simulink library "Radiator_basic"  (R2016b)
settings: Solver=ode45  StartTime=0.0  StopTime=10.0  RelTol=1e-3  EnableMultiTasking=on
libraries: carnot x2, simulink_extras x1
settings Model: Creator=drhf  LastModifiedBy=drhf
settings DataIOCC: LimitDataPoints=on  SaveFormat=Array  SignalLoggingSaveFormat=ModelDataLogs
settings OptimizationCC: ExpressionDepthLimit=2147483647  LifeSpan=inf
settings DebuggingCC: UnderspecifiedInitializationDetection=Classic  MergeDetectMultiDrivingBlocksExec=none  SolverPrmCheckMsg=warning  FcnCallInpInsideContextMsg=warning  StateNameClashWarn=warning  SFUnexpectedBacktrackingDiag=warning  SFNoUnconditionalDefaultTransitionDiag=warning  SFExecutionAtInitializationDiag=none
settings HardwareCC: ProdBitPerPointer=32  ProdBitPerSizeT=32  ProdBitPerPtrDiffT=32  ProdLargestAtomicFloat=None  ProdIntDivRoundTo=Undefined  ProdEndianess=Unspecified  ProdWordSize=32  ProdHWDeviceType=32-bit Generic
settings ModelReferenceCC: PropagateSignalLabelsOutOfModel=off
settings GRTTargetCC: TargetLangStandard=C89/C90 (ANSI)  GeneratePreprocessorConditionals=Disable all  CombineOutputUpdateFcns=off  GRTInterface=on
settings ConfigComp: CovMetricSettings=dw  CovHtmlReporting=on  CovSaveCumulativeToWorkspaceVar=on  CovSaveSingleToWorkspaceVar=on  CovExternalEMLEnable=off

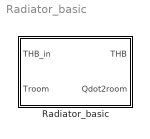
== system Radiator_basic ==
  Radiator_basic : Subsystem  mask(basic Radiator){pnomEN=1000, dtnomEN=50, expo=1.3, mcp=4182*1, tini=20}
      mask prompts: pnomEN "Qdot_nom: nominal power in W"; dtnomEN "Tdiff_nom: nominal temperature difference in K"; expo "radiator exponent (> 0)"; mcp "mass * capacity per unit in J/K"; tini "Initial temperature in °C"
      mask help:
      | The block calculates the heat transfer of a radiator to a room according to the EN 442 equation.
      | Qdot = Qdot_nom * (Tdiff/Tdiff_nom)^n
      mask init:
      | mcap = max(1,mcp); % lower limit for capacity is 1 J/K
      | 
      | % correct values because current model 
      | % uses outlet temperature as mean temperature
      | pnom = pnomEN;
      | dtnom = dtnomEN-5;
      mask Help: web(['file:///' fullfile(path_carnot('help'),'Radiator.html')],'-helpbrowser')

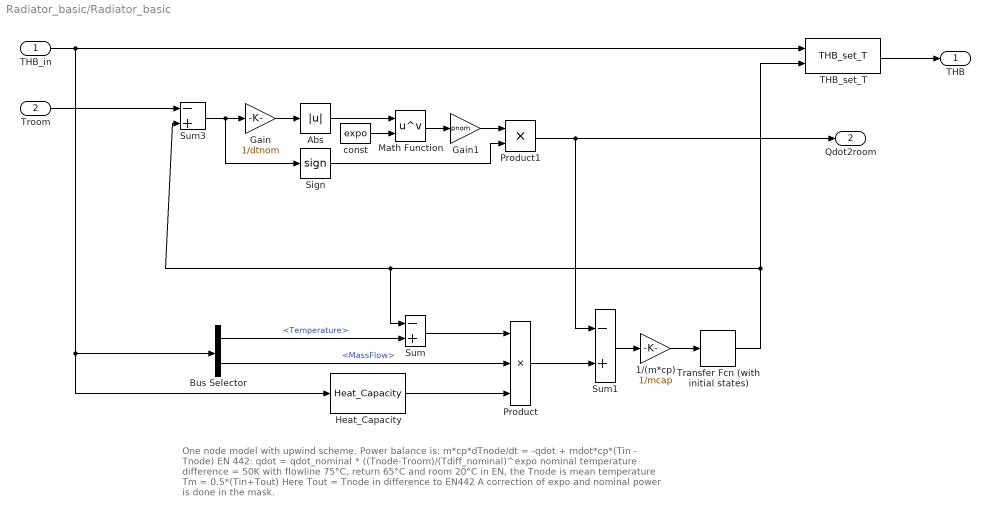
== system Radiator_basic/Radiator_basic ==
  note: One node model with upwind scheme. Power balance is:
      | m*cp*dTnode/dt = -qdot + mdot*cp*(Tin - Tnode)
      |
      | EN 442:
      | qdot = qdot_nominal * ((Tnode-Troom)/(Tdiff_nominal)^expo
      | nominal temperature difference = 50K with flowline 75°C, return 65°C and room 20°C
      | in EN, the Tnode is mean temperature Tm = 0.5*(Tin+Tout)
      |
      | Here Tout = Tnode in difference to EN442
      | A correction of expo and nominal power is done in the mask.
  THB_in : Inport
  Troom : Inport  Port=2
  1/(m*cp) : Gain  Gain=1/mcap  SaturateOnIntegerOverflow=on  OutDataTypeStr=Inherit: Same as input  ParamDataTypeStr=Inherit: Same as input
  Abs : Abs  SaturateOnIntegerOverflow=on
  Bus Selector : BusSelector  OutputSignals=Temperature,MassFlow
  Gain : Gain  Gain=1/dtnom  SaturateOnIntegerOverflow=on  OutDataTypeStr=Inherit: Same as input  ParamDataTypeStr=Inherit: Same as input
  Gain1 : Gain  Gain=pnom  SaturateOnIntegerOverflow=on  OutDataTypeStr=Inherit: Same as input  ParamDataTypeStr=Inherit: Same as input
  Heat_Capacity : carnot/Basic/Material_Properties/Heat_Capacity  VariantControl=CarlibClassic  INPUTARGUMENTS=THB  DEBUGLEVEL=DEBUGLEVEL  MAXTOTALWARNINGS=inf  MAXCONSECUTIVEWARNINGS=inf  WRITETOFILE=0  FILENAME='errors.txt'
  Math Function : Math  Operator=pow  SaturateOnIntegerOverflow=on
  Product : Product  Inputs=3  SaturateOnIntegerOverflow=on  InputSameDT=on  OutDataTypeStr=Inherit: Same as first input
  Product1 : Product  SaturateOnIntegerOverflow=on  InputSameDT=on  OutDataTypeStr=Inherit: Same as first input
  Sign : Signum
  Sum : Sum  Inputs=-+  SaturateOnIntegerOverflow=on  InputSameDT=on  OutDataTypeStr=Inherit: Same as first input
  Sum1 : Sum  Inputs=-+  SaturateOnIntegerOverflow=on  InputSameDT=on  OutDataTypeStr=Inherit: Same as first input
  Sum3 : Sum  Inputs=-+  SaturateOnIntegerOverflow=on  InputSameDT=on  OutDataTypeStr=Inherit: Same as first input
  THB_set_T : carnot/Source/Simple/THB_set_T
  Transfer Fcn (with initial states) : simulink_extras/Additional Linear/Transfer Fcn (with initial states)  N=[1]  D="[1  0]"  X0=tini
  const : Constant  Value=expo
  THB : Outport
  Qdot2room : Outport  Port=2
  wires:
  THB_in/1 -> THB_set_T/1, Heat_Capacity/1, Bus Selector/1
  THB_set_T/1 -> THB/1
  Transfer Fcn (with initial states)/1 -> THB_set_T/2, Sum/1, Sum3/2
  1/(m*cp)/1 -> Transfer Fcn (with initial states)/1
  Sum1/1 -> 1/(m*cp)/1
  Product/1 -> Sum1/2
  Heat_Capacity/1 -> Product/3
  Bus Selector/2 -> Product/2  "<MassFlow>"
  Sum/1 -> Product/1
  Product1/1 -> Sum1/1, Qdot2room/1
  const/1 -> Math Function/2
  Math Function/1 -> Gain1/1
  Gain/1 -> Abs/1
  Abs/1 -> Math Function/1
  Gain1/1 -> Product1/1
  Sum3/1 -> Gain/1, Sign/1
  Sign/1 -> Product1/2
  Bus Selector/1 -> Sum/2  "<Temperature>"
  Troom/1 -> Sum3/1
